simulink model "NoDifferentialControl"  (R2026b)
settings Model: Creator=The MathWorks, Inc.  LastModifiedBy=The MathWorks, Inc.

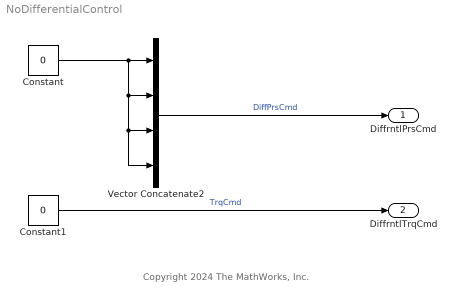
== system NoDifferentialControl ==
  note: Copyright 2024 The MathWorks, Inc.
  Constant : Constant  Value=0  SampleTime=-1
  Constant1 : Constant  Value=0  SampleTime=-1
  Vector Concatenate2 : Concatenate  NumInputs=4
  DiffrntlPrsCmd : Outport  VectorParamsAs1DForOutWhenUnconnected=off
  DiffrntlTrqCmd : Outport  Port=2  VectorParamsAs1DForOutWhenUnconnected=off
  wires:
  Vector Concatenate2/1 -> DiffrntlPrsCmd/1  "DiffPrsCmd"
  Constant1/1 -> DiffrntlTrqCmd/1  "TrqCmd"
  Constant/1 -> Vector Concatenate2/2, Vector Concatenate2/3, Vector Concatenate2/4, Vector Concatenate2/1
